simulink model "pattern3x3_training_2023clock"  (R2024a)
settings: Solver=FixedStepAuto  StartTime=0.0  StopTime=2  FixedStep=0.000005  RelTol=1e-3
model workspace (MAT data in the model file):
  part1_v1 = 1
values from neighbouring files (symbols this model uses):
  full_pattern = load('Pattern4_250.CSV')    [model_setup4.m]
  max_weight2 = 255    [model_setup4.m]
  min_weight2 = 150    [model_setup4.m]
  Th_minus_count2 = 10    [model_setup4.m]    (also in model_setup_test.m = 5)
  Th_plus_count2 = 20    [model_setup4.m]    (also in model_setup_test.m)
libraries: simulink x1
(part 1 of 9)
settings Model: Creator=ITSC  LastModifiedBy=itsc
settings SolverCC: AlgebraicLoopSolver=TrustRegion
settings OptimizationCC: ReuseModelBlockBuffer=off
settings DebuggingCC: UnconnectedInputMsg=warning  UnconnectedOutputMsg=warning  UnconnectedLineMsg=warning
settings ModelReferenceCC: EnableRefExpFcnMdlSchedulingChecks=on
settings RTWCC: GPUComputeCapability=3.5  DLArmComputeVersion=19.05

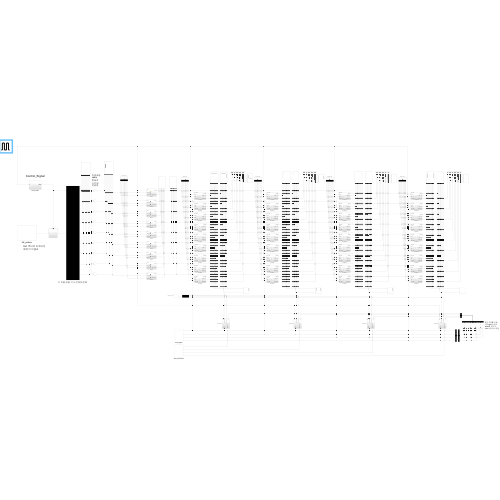
[thumbnail: Simulink's stored preview of the top-level diagram]
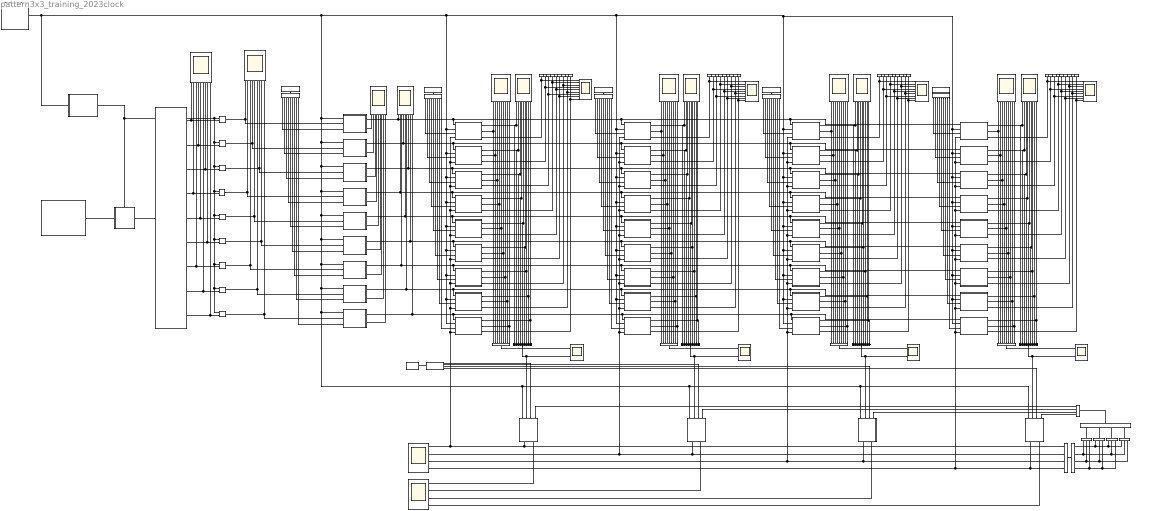
== system pattern3x3_training_2023clock ==
  note: 픽셀값을 spike 형태로 뉴런에 전달함
  note: 각 픽셀 값을 각 뉴런에게 분배
  note: 9x1 벡터로 이루어진 패턴의 픽셀값
  note: 측면 억제를 위해 다른 post 뉴런의 spike를 모아 각 post 뉴런으로 전달
  note: Control_Signal
  Bus Creator : BusCreator  Inputs=4
  Bus Creator1 : BusCreator  Inputs=4
  Bus Selector : BusSelector  OutputSignals=signal1,signal2,signal3,signal4
  Bus Selector1 : BusSelector  OutputSignals=signal1,signal2,signal3,signal4
  Demux{1..6} (6 alike) : Demux  Outputs=9
  Demux7 : Demux
  Neuron1 : Subsystem
  Neuron2 : Subsystem
  Neuron3 : Subsystem
  Neuron4 : Subsystem
  Neuron5 : Subsystem
  Neuron6 : Subsystem
  Neuron7 : Subsystem
  Neuron8 : Subsystem
  Neuron9 : Subsystem
  OR{,1..3} (4 alike) : Logic  Operator=OR  Inputs=3  IconShape=distinctive  AllPortsSameDT=off  OutDataTypeStr=boolean
  OR{8..11} (4 alike) : Logic  Operator=OR  Inputs=9  AllPortsSameDT=off  OutDataTypeStr=boolean
  Post_Neuron1 : Subsystem
  Post_Neuron2 : Subsystem
  Post_Neuron3 : Subsystem
  Post_Neuron4 : Subsystem
  Post_Spike : Scope  NumInputPorts=4
  Post_Threshold : Scope  NumInputPorts=4
  Product{1..9} (9 alike) : Product
  Pulse Generator2 : DiscretePulseGenerator  PulseType=Time based  Period=0.0001  PulseWidth=50
  Scope{,1..14,19} (16 alike) : Scope  NumInputPorts=9
  Scope{15..18} (4 alike) : Scope  NumInputPorts=2
  Subsystem1 : Subsystem
  Sum{4..7} (4 alike) : Sum  Inputs=|+++++++++
  Synapse1 : Subsystem
  Synapse10 : Subsystem
  Synapse11 : Subsystem
  Synapse12 : Subsystem
  Synapse13 : Subsystem
  Synapse14 : Subsystem
  Synapse15 : Subsystem
  Synapse16 : Subsystem
  Synapse17 : Subsystem
  Synapse18 : Subsystem
  Synapse19 : Subsystem
  Synapse2 : Subsystem
  Synapse20 : Subsystem
  Synapse21 : Subsystem
  Synapse22 : Subsystem
  Synapse23 : Subsystem
  Synapse24 : Subsystem
  Synapse25 : Subsystem
  Synapse26 : Subsystem
  Synapse27 : Subsystem
  Synapse28 : Subsystem
  Synapse29 : Subsystem
  Synapse3 : Subsystem
  Synapse30 : Subsystem
  Synapse31 : Subsystem
  Synapse32 : Subsystem
  Synapse33 : Subsystem
  Synapse34 : Subsystem
  Synapse35 : Subsystem
  Synapse36 : Subsystem
  Synapse4 : Subsystem
  Synapse5 : Subsystem
  Synapse6 : Subsystem
  Synapse7 : Subsystem
  Synapse8 : Subsystem
  Synapse9 : Subsystem
  To Workspace2 : ToWorkspace  VariableName=w1_2  SampleTime=-1
  To Workspace3 : ToWorkspace  VariableName=w2_2  SampleTime=-1
  To Workspace36 : ToWorkspace  VariableName=w1_1  SampleTime=-1
  To Workspace37 : ToWorkspace  VariableName=w2_1  SampleTime=-1
  To Workspace38 : ToWorkspace  VariableName=w3_1  SampleTime=-1
  To Workspace39 : ToWorkspace  VariableName=w4_1  SampleTime=-1
  To Workspace4 : ToWorkspace  VariableName=w3_2  SampleTime=-1
  To Workspace40 : ToWorkspace  VariableName=w5_1  SampleTime=-1
  To Workspace41 : ToWorkspace  VariableName=w6_1  SampleTime=-1
  To Workspace42 : ToWorkspace  VariableName=w7_1  SampleTime=-1
  To Workspace43 : ToWorkspace  VariableName=w8_1  SampleTime=-1
  To Workspace44 : ToWorkspace  VariableName=w9_1  SampleTime=-1
  To Workspace45 : ToWorkspace  VariableName=w9_2  SampleTime=-1
  To Workspace46 : ToWorkspace  VariableName=w1_3  SampleTime=-1
  To Workspace47 : ToWorkspace  VariableName=w2_3  SampleTime=-1
  To Workspace48 : ToWorkspace  VariableName=w3_3  SampleTime=-1
  To Workspace49 : ToWorkspace  VariableName=w4_3  SampleTime=-1
  To Workspace5 : ToWorkspace  VariableName=w4_2  SampleTime=-1
  To Workspace50 : ToWorkspace  VariableName=w5_3  SampleTime=-1
  To Workspace51 : ToWorkspace  VariableName=w6_3  SampleTime=-1
  To Workspace52 : ToWorkspace  VariableName=w7_3  SampleTime=-1
  To Workspace53 : ToWorkspace  VariableName=w8_3  SampleTime=-1
  To Workspace54 : ToWorkspace  VariableName=w9_3  SampleTime=-1
  To Workspace55 : ToWorkspace  VariableName=w1_4  SampleTime=-1
  To Workspace56 : ToWorkspace  VariableName=w2_4  SampleTime=-1
  To Workspace57 : ToWorkspace  VariableName=w3_4  SampleTime=-1
  To Workspace58 : ToWorkspace  VariableName=w4_4  SampleTime=-1
  To Workspace59 : ToWorkspace  VariableName=w5_4  SampleTime=-1
  To Workspace6 : ToWorkspace  VariableName=w5_2  SampleTime=-1
  To Workspace60 : ToWorkspace  VariableName=w6_4  SampleTime=-1
  To Workspace61 : ToWorkspace  VariableName=w7_4  SampleTime=-1
  To Workspace62 : ToWorkspace  VariableName=w8_4  SampleTime=-1
  To Workspace63 : ToWorkspace  VariableName=w9_4  SampleTime=-1
  To Workspace7 : ToWorkspace  VariableName=w6_2  SampleTime=-1
  To Workspace8 : ToWorkspace  VariableName=w7_2  SampleTime=-1
  To Workspace9 : ToWorkspace  VariableName=w8_2  SampleTime=-1
  clock_0.001 : Subsystem
  full_pattern : Constant  Value=full_pattern
  post_neuron_num : Constant  Value=[1 2 3 4]  VectorParams1D=off
  pre_neuron_num : Constant  Value=[1 2 3 4 5 6 7 8 9]  VectorParams1D=off
  synapse_num1 : Constant  Value=[1 2 3 4 5 6 7 8 9]  VectorParams1D=off
  synapse_num2 : Constant  Value=[10 11 12 13 14 15 16 17 18]  VectorParams1D=off
  synapse_num3 : Constant  Value=[19 20 21 22 23 24 25 26 27]  VectorParams1D=off
  synapse_num4 : Constant  Value=[28 29 30 31 32 33 34 35 36]  VectorParams1D=off
  wires:
  Demux1/4 -> Product3/2, Scope/2
  Demux1/5 -> Product4/2, Scope/5
  Demux1/2 -> Product1/2, Scope/4
  Demux1/6 -> Product5/2, Scope/8
  Demux1/8 -> Product7/2, Scope/6
  Subsystem1/1(y) -> Demux1/1
  Demux1/7 -> Product6/2, Scope/3
  Demux1/3 -> Product2/2, Scope/7
  Demux1/9 -> Product8/2, Scope/9
  Neuron1/1("Spike ") -> Synapse1/1(Pre_spike), Synapse10/1(Pre_spike), Synapse28/1(Pre_spike), Synapse19/1(Pre_spike), Scope9/1
  Neuron3/1("Spike ") -> Scope9/7, Synapse3/1(Pre_spike), Synapse12/1(Pre_spike), Synapse30/1(Pre_spike), Synapse21/1(Pre_spike)
  Neuron4/1("Spike ") -> Scope9/2, Synapse4/1(Pre_spike), Synapse13/1(Pre_spike), Synapse31/1(Pre_spike), Synapse22/1(Pre_spike)
  Neuron5/1("Spike ") -> Scope9/5, Synapse5/1(Pre_spike), Synapse14/1(Pre_spike), Synapse32/1(Pre_spike), Synapse23/1(Pre_spike)
  Neuron6/1("Spike ") -> Scope9/8, Synapse6/1(Pre_spike), Synapse15/1(Pre_spike), Synapse33/1(Pre_spike), Synapse24/1(Pre_spike)
  Neuron7/1("Spike ") -> Scope9/3, Synapse7/1(Pre_spike), Synapse16/1(Pre_spike), Synapse34/1(Pre_spike), Synapse25/1(Pre_spike)
  Neuron8/1("Spike ") -> Scope9/6, Synapse8/1(Pre_spike), Synapse17/1(Pre_spike), Synapse35/1(Pre_spike), Synapse26/1(Pre_spike)
  Neuron9/1("Spike ") -> Scope9/9, Synapse9/1(Pre_spike), Synapse18/1(Pre_spike), Synapse36/1(Pre_spike), Synapse27/1(Pre_spike)
  Neuron2/1("Spike ") -> Synapse2/1(Pre_spike), Synapse11/1(Pre_spike), Synapse29/1(Pre_spike), Synapse20/1(Pre_spike), Scope9/4
  OR8/1 -> Scope15/1
  Sum5/1 -> Post_Neuron1/2(Input_potential), Scope15/2
  Synapse8/2(Spike_out) -> Scope4/8, OR8/8
  Synapse7/2(Spike_out) -> Scope4/7, OR8/7
  Synapse6/2(Spike_out) -> Scope4/6, OR8/6
  Synapse4/1(Weight) -> Scope8/4, Sum5/4
  Synapse4/2(Spike_out) -> Scope4/4, OR8/4
  Synapse3/1(Weight) -> Scope8/3, Sum5/3
  Synapse3/2(Spike_out) -> Scope4/3, OR8/3
  Synapse2/2(Spike_out) -> Scope4/2, OR8/2
  Synapse9/2(Spike_out) -> Scope4/9, OR8/9
  Synapse1/2(Spike_out) -> Scope4/1, OR8/1
  Synapse5/2(Spike_out) -> Scope4/5, OR8/5
  Synapse7/1(Weight) -> Scope8/7, Sum5/7
  Synapse8/1(Weight) -> Scope8/8, Sum5/8
  Synapse9/1(Weight) -> Scope8/9, Sum5/9
  Neuron1/2(threshold_view) -> Scope7/1
  Neuron2/2(threshold_view) -> Scope7/2
  Neuron3/2(threshold_view) -> Scope7/3
  Neuron4/2(threshold_view) -> Scope7/4
  Neuron5/2(threshold_view) -> Scope7/5
  Neuron6/2(threshold_view) -> Scope7/6
  Neuron7/2(threshold_view) -> Scope7/7
  Neuron8/2(threshold_view) -> Scope7/8
  Neuron9/2(threshold_view) -> Scope7/9
  synapse_num1/1 -> Demux2/1
  Synapse5/1(Weight) -> Scope8/5, Sum5/5
  Synapse6/1(Weight) -> Scope8/6, Sum5/6
  Demux2/1 -> Synapse1/3(addr)
  Demux2/2 -> Synapse2/3(addr)
  Demux2/3 -> Synapse3/3(addr)
  Demux2/4 -> Synapse4/3(addr)
  Demux2/5 -> Synapse5/3(addr)
  Demux2/6 -> Synapse6/3(addr)
  Demux2/7 -> Synapse7/3(addr)
  Demux2/8 -> Synapse8/3(addr)
  Demux2/9 -> Synapse9/3(addr)
  Demux3/5 -> Synapse14/3(addr)
  Demux3/1 -> Synapse10/3(addr)
  Demux3/6 -> Synapse15/3(addr)
  Demux3/7 -> Synapse16/3(addr)
  Demux3/8 -> Synapse17/3(addr)
  Demux3/2 -> Synapse11/3(addr)
  Demux3/3 -> Synapse12/3(addr)
  Demux3/4 -> Synapse13/3(addr)
  Demux3/9 -> Synapse18/3(addr)
  synapse_num2/1 -> Demux3/1
  Demux4/1 -> Synapse19/3(addr)
  Demux4/8 -> Synapse26/3(addr)
  Demux4/7 -> Synapse25/3(addr)
  synapse_num3/1 -> Demux4/1
  Demux4/2 -> Synapse20/3(addr)
  Demux4/5 -> Synapse23/3(addr)
  Demux4/9 -> Synapse27/3(addr)
  Demux4/4 -> Synapse22/3(addr)
  Demux4/3 -> Synapse21/3(addr)
  Demux4/6 -> Synapse24/3(addr)
  Demux5/5 -> Synapse32/3(addr)
  Demux5/1 -> Synapse28/3(addr)
  Demux5/6 -> Synapse33/3(addr)
  Demux5/7 -> Synapse34/3(addr)
  Demux5/8 -> Synapse35/3(addr)
  Demux5/2 -> Synapse29/3(addr)
  Demux5/3 -> Synapse30/3(addr)
  Demux5/4 -> Synapse31/3(addr)
  Demux5/9 -> Synapse36/3(addr)
  synapse_num4/1 -> Demux5/1
  Post_Neuron1/1(Spike) -> Synapse9/4(Post_spike), Synapse8/4(Post_spike), Synapse7/4(Post_spike), Synapse6/4(Post_spike), Synapse5/4(Post_spike), Synapse4/4(Post_spike), Synapse3/4(Post_spike), Synapse2/4(Post_spike), Synapse1/4(Post_spike), Post_Spike/1, Bus Creator/1
  Post_Neuron2/1(Spike) -> Synapse18/4(Post_spike), Synapse17/4(Post_spike), Synapse16/4(Post_spike), Synapse15/4(Post_spike), Synapse14/4(Post_spike), Synapse13/4(Post_spike), Synapse12/4(Post_spike), Synapse11/4(Post_spike), Synapse10/4(Post_spike), Post_Spike/2, Bus Creator/2
  Post_Neuron3/1(Spike) -> Synapse27/4(Post_spike), Synapse26/4(Post_spike), Synapse25/4(Post_spike), Synapse24/4(Post_spike), Synapse23/4(Post_spike), Synapse22/4(Post_spike), Synapse21/4(Post_spike), Synapse19/4(Post_spike), Synapse20/4(Post_spike), Post_Spike/3, Bus Creator/3
  Post_Neuron1/2(threshold_view) -> Post_Threshold/1
  Post_Neuron2/2(threshold_view) -> Post_Threshold/2
  Post_Neuron3/2(threshold_view) -> Post_Threshold/3
  Post_Neuron4/2(threshold_view) -> Post_Threshold/4
  Post_Neuron4/1(Spike) -> Synapse36/4(Post_spike), Synapse35/4(Post_spike), Synapse34/4(Post_spike), Synapse33/4(Post_spike), Synapse32/4(Post_spike), Synapse31/4(Post_spike), Synapse30/4(Post_spike), Synapse29/4(Post_spike), Synapse28/4(Post_spike), Post_Spike/4, Bus Creator/4
  Synapse6/3(Weight_out) -> Scope11/8, To Workspace41/1
  Synapse9/3(Weight_out) -> Scope11/9, To Workspace44/1
  Synapse7/3(Weight_out) -> Scope11/3, To Workspace42/1
  Synapse1/3(Weight_out) -> Scope11/1, To Workspace36/1
  Synapse4/3(Weight_out) -> Scope11/2, To Workspace39/1
  Synapse8/3(Weight_out) -> Scope11/6, To Workspace43/1
  Synapse2/3(Weight_out) -> Scope11/4, To Workspace37/1
  Synapse3/3(Weight_out) -> Scope11/7, To Workspace38/1
  Synapse15/2(Spike_out) -> Scope5/6, OR9/6
  Synapse12/2(Spike_out) -> Scope5/3, OR9/3
  Synapse18/2(Spike_out) -> Scope5/9, OR9/9
  Synapse13/2(Spike_out) -> Scope5/4, OR9/4
  Synapse10/2(Spike_out) -> Scope5/1, OR9/1
  Synapse11/2(Spike_out) -> Scope5/2, OR9/2
  Synapse16/2(Spike_out) -> Scope5/7, OR9/7
  Synapse14/2(Spike_out) -> Scope5/5, OR9/5
  Synapse17/2(Spike_out) -> Scope5/8, OR9/8
  Synapse24/2(Spike_out) -> Scope6/6, OR10/6
  Synapse21/2(Spike_out) -> Scope6/3, OR10/3
  Synapse27/2(Spike_out) -> Scope6/9, OR10/9
  Synapse22/2(Spike_out) -> Scope6/4, OR10/4
  Synapse19/2(Spike_out) -> Scope6/1, OR10/1
  Synapse20/2(Spike_out) -> Scope6/2, OR10/2
  Synapse25/2(Spike_out) -> Scope6/7, OR10/7
  Synapse23/2(Spike_out) -> Scope6/5, OR10/5
  Synapse26/2(Spike_out) -> Scope6/8, OR10/8
  Synapse33/2(Spike_out) -> Scope10/6, OR11/6
  Synapse30/2(Spike_out) -> Scope10/3, OR11/3
  Synapse36/2(Spike_out) -> Scope10/9, OR11/9
  Synapse31/2(Spike_out) -> Scope10/4, OR11/4
  Synapse28/2(Spike_out) -> Scope10/1, OR11/1
  Synapse29/2(Spike_out) -> Scope10/2, OR11/2
  Synapse34/2(Spike_out) -> Scope10/7, OR11/7
  Synapse32/2(Spike_out) -> Scope10/5, OR11/5
  Synapse35/2(Spike_out) -> Scope10/8, OR11/8
  Synapse5/3(Weight_out) -> Scope11/5, To Workspace40/1
  Synapse16/3(Weight_out) -> Scope12/3, To Workspace8/1
  Synapse12/3(Weight_out) -> Scope12/7, To Workspace4/1
  Synapse11/3(Weight_out) -> Scope12/4, To Workspace3/1
  Synapse15/3(Weight_out) -> Scope12/8, To Workspace7/1
  Synapse14/3(Weight_out) -> Scope12/5, To Workspace6/1
  Synapse13/3(Weight_out) -> Scope12/2, To Workspace5/1
  Synapse17/3(Weight_out) -> Scope12/6, To Workspace9/1
  Synapse10/3(Weight_out) -> Scope12/1, To Workspace2/1
  Synapse18/3(Weight_out) -> Scope12/9, To Workspace45/1
  Synapse25/3(Weight_out) -> Scope13/3, To Workspace52/1
  Synapse21/3(Weight_out) -> Scope13/7, To Workspace48/1
  Synapse20/3(Weight_out) -> Scope13/4, To Workspace47/1
  Synapse24/3(Weight_out) -> Scope13/8, To Workspace51/1
  Synapse23/3(Weight_out) -> To Workspace50/1, Scope13/5
  Synapse22/3(Weight_out) -> Scope13/2, To Workspace49/1
  Synapse26/3(Weight_out) -> Scope13/6, To Workspace53/1
  Synapse19/3(Weight_out) -> To Workspace46/1, Scope13/1
  Synapse27/3(Weight_out) -> To Workspace54/1, Scope13/9
  Synapse34/3(Weight_out) -> Scope14/3, To Workspace61/1
  Synapse30/3(Weight_out) -> Scope14/7, To Workspace57/1
  Synapse29/3(Weight_out) -> Scope14/4, To Workspace56/1
  Synapse33/3(Weight_out) -> Scope14/8, To Workspace60/1
  Synapse32/3(Weight_out) -> Scope14/5, To Workspace59/1
  Synapse31/3(Weight_out) -> Scope14/2, To Workspace58/1
  Synapse35/3(Weight_out) -> Scope14/6, To Workspace62/1
  Synapse28/3(Weight_out) -> Scope14/1, To Workspace55/1
  Synapse36/3(Weight_out) -> Scope14/9, To Workspace63/1
  OR9/1 -> Scope16/1
  Sum4/1 -> Post_Neuron2/2(Input_potential), Scope16/2
  OR10/1 -> Scope17/1
  Sum6/1 -> Post_Neuron3/2(Input_potential), Scope17/2
  Sum7/1 -> Post_Neuron4/2(Input_potential), Scope18/2
  OR11/1 -> Scope18/1
  Synapse1/1(Weight) -> Scope8/1, Sum5/1
  Synapse2/1(Weight) -> Scope8/2, Sum5/2
  Synapse14/1(Weight) -> Scope1/5, Sum4/5
  Synapse12/1(Weight) -> Scope1/3, Sum4/3
  Synapse13/1(Weight) -> Scope1/4, Sum4/4
  Synapse10/1(Weight) -> Scope1/1, Sum4/1
  Synapse15/1(Weight) -> Scope1/6, Sum4/6
  Synapse18/1(Weight) -> Scope1/9, Sum4/9
  Synapse17/1(Weight) -> Scope1/8, Sum4/8
  Synapse16/1(Weight) -> Scope1/7, Sum4/7
  Synapse11/1(Weight) -> Scope1/2, Sum4/2
  Synapse23/1(Weight) -> Scope2/5, Sum6/5
  Synapse21/1(Weight) -> Scope2/3, Sum6/3
  Synapse22/1(Weight) -> Scope2/4, Sum6/4
  Synapse19/1(Weight) -> Scope2/1, Sum6/1
  Synapse24/1(Weight) -> Scope2/6, Sum6/6
  Synapse27/1(Weight) -> Scope2/9, Sum6/9
  Synapse26/1(Weight) -> Scope2/8, Sum6/8
  Synapse25/1(Weight) -> Scope2/7, Sum6/7
  Synapse20/1(Weight) -> Scope2/2, Sum6/2
  Synapse32/1(Weight) -> Scope3/5, Sum7/5
  Synapse30/1(Weight) -> Scope3/3, Sum7/3
  Synapse31/1(Weight) -> Scope3/4, Sum7/4
  Synapse28/1(Weight) -> Scope3/1, Sum7/1
  Synapse33/1(Weight) -> Scope3/6, Sum7/6
  Synapse36/1(Weight) -> Scope3/9, Sum7/9
  Synapse35/1(Weight) -> Scope3/8, Sum7/8
  Synapse34/1(Weight) -> Scope3/7, Sum7/7
  Synapse29/1(Weight) -> Scope3/2, Sum7/2
  clock_0.001/1(clock) -> Subsystem1/Trigger, Product3/1, Product4/1, Product8/1, Product7/1, Product6/1, Product5/1, Product2/1, Product1/1, Product9/1
  Demux1/1 -> Product9/2, Scope/1
  Demux6/5 -> Neuron5/3(neuron_num)
  Demux6/6 -> Neuron6/3(neuron_num)
  Demux6/7 -> Neuron7/3(neuron_num)
  Demux6/4 -> Neuron4/3(neuron_num)
  Demux6/3 -> Neuron3/3(neuron_num)
  Demux6/2 -> Neuron2/3(neuron_num)
  Demux6/9 -> Neuron9/3(neuron_num)
  Demux6/8 -> Neuron8/3(neuron_num)
  Demux6/1 -> Neuron1/3(neuron_num)
  pre_neuron_num/1 -> Demux6/1
  post_neuron_num/1 -> Demux7/1
  Demux7/1 -> Post_Neuron1/3(neuron_num)
  Demux7/2 -> Post_Neuron2/3(neuron_num)
  Demux7/3 -> Post_Neuron3/3(neuron_num)
  Demux7/4 -> Post_Neuron4/3(neuron_num)
  Bus Creator/1 -> Bus Selector/1
  Bus Selector/2 -> OR3/2, OR2/2, OR/1  "<signal2>"
  Bus Selector/3 -> OR3/3, OR1/2, OR/2  "<signal3>"
  Bus Selector/4 -> OR2/3, OR1/3, OR/3  "<signal4>"
  Bus Selector/1 -> OR3/1, OR2/1, OR1/1  "<signal1>"
  OR/1 -> Bus Creator1/1
  OR3/1 -> Bus Creator1/4
  OR2/1 -> Bus Creator1/3
  OR1/1 -> Bus Creator1/2
  Bus Creator1/1 -> Bus Selector1/1
  Bus Selector1/1 -> Post_Neuron1/4(wta)  "<signal1>"
  Bus Selector1/2 -> Post_Neuron2/4(wta)  "<signal2>"
  Bus Selector1/3 -> Post_Neuron3/4(wta)  "<signal3>"
  Bus Selector1/4 -> Post_Neuron4/4(wta)  "<signal4>"
  full_pattern/1 -> Subsystem1/1(data)
  Product1/1 -> Neuron2/2(Input_potential), Scope19/4
  Product5/1 -> Neuron6/2(Input_potential), Scope19/8
  Product2/1 -> Neuron3/2(Input_potential), Scope19/7
  Product4/1 -> Neuron5/2(Input_potential), Scope19/5
  Product7/1 -> Neuron8/2(Input_potential), Scope19/6
  Product3/1 -> Neuron4/2(Input_potential), Scope19/2
  Product6/1 -> Neuron7/2(Input_potential), Scope19/3
  Product8/1 -> Neuron9/2(Input_potential), Scope19/9
  Product9/1 -> Neuron1/2(Input_potential), Scope19/1
  Pulse Generator2/1 -> clock_0.001/1(In1), Neuron1/1(clock), Neuron2/1(clock), Neuron3/1(clock), Neuron4/1(clock), Neuron5/1(clock), Neuron6/1(clock), Neuron7/1(clock), Neuron8/1(clock), Neuron9/1(clock), Post_Neuron2/1(clock), Post_Neuron4/1(clock), Post_Neuron3/1(clock), Post_Neuron1/1(clock), Synapse28/2(clock), Synapse29/2(clock), Synapse30/2(clock), Synapse31/2(clock), Synapse32/2(clock), Synapse33/2(clock), Synapse34/2(clock), Synapse36/2(clock), Synapse35/2(clock), Synapse19/2(clock), Synapse20/2(clock), Synapse21/2(clock), Synapse22/2(clock), Synapse23/2(clock), Synapse24/2(clock), Synapse25/2(clock), Synapse27/2(clock), Synapse26/2(clock), Synapse10/2(clock), Synapse11/2(clock), Synapse12/2(clock), Synapse13/2(clock), Synapse14/2(clock), Synapse15/2(clock), Synapse16/2(clock), Synapse18/2(clock), Synapse17/2(clock), Synapse2/2(clock), Synapse3/2(clock), Synapse4/2(clock), Synapse5/2(clock), Synapse6/2(clock), Synapse7/2(clock), Synapse9/2(clock), Synapse8/2(clock), Synapse1/2(clock)

== system pattern3x3_training_2023clock/Neuron1 ==
  note: Membrane potential part
  note: Input potential이 추가로 들어오기 전에는 이전
      | membrane state를 유지해야 하기 때문에 Trigger 사용
  note: Output 스파이크 빈도에 따라 Threshold 조절
  note: membrane potential>=threshold
  note: membrane potential
      | - threshold
  note: 뉴런 번호
  note: membrane potential<threshold
  note: membrane potential - threshold >= 0 일때 spike=1
  note: Threshold part
  note: Spike part
  note: membrane state
      | - threshold
  clock : Inport
  Input_potential : Inport  Port=2  OutDataTypeStr=double
  neuron_num : Inport  Port=3  OutDataTypeStr=double
  Clock4 : Subsystem
  Delay : Delay  DelayLength=1  InitialCondition=0
  From Workspace4 : FromWorkspace  VariableName=threshold_pre
  MATLAB Function3 : MATLAB Function  TreatAsAtomicUnit=on
  MATLAB Function4 : MATLAB Function  TreatAsAtomicUnit=on
  MATLAB Function5 : MATLAB Function  TreatAsAtomicUnit=on
  Memory2 : Memory
  Scope4 : Scope  NumInputPorts=5
  Scope9 : Scope  NumInputPorts=6
  Subsystem2 : Subsystem
  Subsystem3 : Subsystem
  Subtract2 : Sum  Inputs=+-
  Subtract3 : Sum  Inputs=+-
  Switch1 : Switch  SaturateOnIntegerOverflow=off  InputSameDT=off
  spike_generator1 : Subsystem
  "Spike " : Outport  VectorParamsAs1DForOutWhenUnconnected=off
  threshold_view : Outport  Port=2
  wires:
  Switch1/1 -> Delay/1, Subtract2/1, Scope9/1
  Subtract2/1 -> Scope9/3, MATLAB Function3/1(u)
  MATLAB Function3/1(y) -> Memory2/1, Scope9/4
  Clock4/1(T) -> Scope4/3, MATLAB Function5/1(t), MATLAB Function4/2(t)
  Subsystem3/1(Threshold) -> Subtract2/2, Scope9/2, Subtract3/2, threshold_view/1
  neuron_num/1 -> Subsystem3/3(neuron_num)
  From Workspace4/1 -> Subsystem3/2(initial_threshold)
  MATLAB Function5/1(membrane_potential) -> Scope4/4, Switch1/1
  MATLAB Function4/1(membrane_potential) -> Switch1/3, Scope4/5
  Subsystem2/1(membrane_state) -> MATLAB Function4/1(membrane_state), Subtract3/1, Scope4/2, MATLAB Function5/2(membrane_state)
  spike_generator1/1(spike) -> "Spike "/1, Scope9/6, Subsystem3/1(spike)
  Input_potential/1 -> Subsystem2/1(Input potential), Subsystem2/Trigger, Scope4/1, Clock4/2("Reset ")
  Subtract3/1 -> Switch1/2
  Memory2/1 -> Scope9/5, spike_generator1/1(1)
  Delay/1 -> Subsystem2/2(before_Potential)
  clock/1 -> Subsystem3/4(clock), Clock4/1(clock)

== system pattern3x3_training_2023clock/Neuron2 ==
  note: Membrane potential part
  note: Input potential이 추가로 들어오기 전에는 이전
      | membrane state를 유지해야 하기 때문에 Trigger 사용
  note: Output 스파이크 빈도에 따라 Threshold 조절
  note: membrane potential>=threshold
  note: membrane potential
      | - threshold
  note: 뉴런 번호
  note: membrane potential<threshold
  note: membrane potential - threshold >= 0 일때 spike=1
  note: Threshold part
  note: Spike part
  note: membrane state
      | - threshold
  clock : Inport
  Input_potential : Inport  Port=2  OutDataTypeStr=double
  neuron_num : Inport  Port=3  OutDataTypeStr=double
  Clock4 : Subsystem
  Delay : Delay  DelayLength=1  InitialCondition=0
  From Workspace4 : FromWorkspace  VariableName=threshold_pre
  MATLAB Function3 : MATLAB Function  TreatAsAtomicUnit=on
  MATLAB Function4 : MATLAB Function  TreatAsAtomicUnit=on
  MATLAB Function5 : MATLAB Function  TreatAsAtomicUnit=on
  Memory2 : Memory
  Scope4 : Scope  NumInputPorts=5
  Scope9 : Scope  NumInputPorts=6
  Subsystem2 : Subsystem
  Subsystem3 : Subsystem
  Subtract2 : Sum  Inputs=+-
  Subtract3 : Sum  Inputs=+-
  Switch1 : Switch  SaturateOnIntegerOverflow=off  InputSameDT=off
  spike_generator1 : Subsystem
  "Spike " : Outport  VectorParamsAs1DForOutWhenUnconnected=off
  threshold_view : Outport  Port=2
  wires:
  Switch1/1 -> Delay/1, Subtract2/1, Scope9/1
  Subtract2/1 -> Scope9/3, MATLAB Function3/1(u)
  MATLAB Function3/1(y) -> Memory2/1, Scope9/4
  Clock4/1(T) -> Scope4/3, MATLAB Function5/1(t), MATLAB Function4/2(t)
  Subsystem3/1(Threshold) -> Subtract2/2, Scope9/2, Subtract3/2, threshold_view/1
  neuron_num/1 -> Subsystem3/3(neuron_num)
  From Workspace4/1 -> Subsystem3/2(initial_threshold)
  MATLAB Function5/1(membrane_potential) -> Scope4/4, Switch1/1
  MATLAB Function4/1(membrane_potential) -> Switch1/3, Scope4/5
  Subsystem2/1(membrane_state) -> MATLAB Function4/1(membrane_state), Subtract3/1, Scope4/2, MATLAB Function5/2(membrane_state)
  spike_generator1/1(spike) -> "Spike "/1, Scope9/6, Subsystem3/1(spike)
  Input_potential/1 -> Subsystem2/1(Input potential), Subsystem2/Trigger, Scope4/1, Clock4/2("Reset ")
  Subtract3/1 -> Switch1/2
  Memory2/1 -> Scope9/5, spike_generator1/1(1)
  Delay/1 -> Subsystem2/2(before_Potential)
  clock/1 -> Subsystem3/4(clock), Clock4/1(clock)

== system pattern3x3_training_2023clock/Neuron3 ==
  note: Membrane potential part
  note: Input potential이 추가로 들어오기 전에는 이전
      | membrane state를 유지해야 하기 때문에 Trigger 사용
  note: Output 스파이크 빈도에 따라 Threshold 조절
  note: membrane potential>=threshold
  note: membrane potential
      | - threshold
  note: 뉴런 번호
  note: membrane potential<threshold
  note: membrane potential - threshold >= 0 일때 spike=1
  note: Threshold part
  note: Spike part
  note: membrane state
      | - threshold
  clock : Inport
  Input_potential : Inport  Port=2  OutDataTypeStr=double
  neuron_num : Inport  Port=3  OutDataTypeStr=double
  Clock4 : Subsystem
  Delay : Delay  DelayLength=1  InitialCondition=0
  From Workspace4 : FromWorkspace  VariableName=threshold_pre
  MATLAB Function3 : MATLAB Function  TreatAsAtomicUnit=on
  MATLAB Function4 : MATLAB Function  TreatAsAtomicUnit=on
  MATLAB Function5 : MATLAB Function  TreatAsAtomicUnit=on
  Memory2 : Memory
  Scope4 : Scope  NumInputPorts=5
  Scope9 : Scope  NumInputPorts=6
  Subsystem2 : Subsystem
  Subsystem3 : Subsystem
  Subtract2 : Sum  Inputs=+-
  Subtract3 : Sum  Inputs=+-
  Switch1 : Switch  SaturateOnIntegerOverflow=off  InputSameDT=off
  spike_generator1 : Subsystem
  "Spike " : Outport  VectorParamsAs1DForOutWhenUnconnected=off
  threshold_view : Outport  Port=2
  wires:
  Switch1/1 -> Delay/1, Subtract2/1, Scope9/1
  Subtract2/1 -> Scope9/3, MATLAB Function3/1(u)
  MATLAB Function3/1(y) -> Memory2/1, Scope9/4
  Clock4/1(T) -> Scope4/3, MATLAB Function5/1(t), MATLAB Function4/2(t)
  Subsystem3/1(Threshold) -> Subtract2/2, Scope9/2, Subtract3/2, threshold_view/1
  neuron_num/1 -> Subsystem3/3(neuron_num)
  From Workspace4/1 -> Subsystem3/2(initial_threshold)
  MATLAB Function5/1(membrane_potential) -> Scope4/4, Switch1/1
  MATLAB Function4/1(membrane_potential) -> Switch1/3, Scope4/5
  Subsystem2/1(membrane_state) -> MATLAB Function4/1(membrane_state), Subtract3/1, Scope4/2, MATLAB Function5/2(membrane_state)
  spike_generator1/1(spike) -> "Spike "/1, Scope9/6, Subsystem3/1(spike)
  Input_potential/1 -> Subsystem2/1(Input potential), Subsystem2/Trigger, Scope4/1, Clock4/2("Reset ")
  Subtract3/1 -> Switch1/2
  Memory2/1 -> Scope9/5, spike_generator1/1(1)
  Delay/1 -> Subsystem2/2(before_Potential)
  clock/1 -> Subsystem3/4(clock), Clock4/1(clock)

== system pattern3x3_training_2023clock/Neuron4 ==
  note: Membrane potential part
  note: Input potential이 추가로 들어오기 전에는 이전
      | membrane state를 유지해야 하기 때문에 Trigger 사용
  note: Output 스파이크 빈도에 따라 Threshold 조절
  note: membrane potential>=threshold
  note: membrane potential
      | - threshold
  note: 뉴런 번호
  note: membrane potential<threshold
  note: membrane potential - threshold >= 0 일때 spike=1
  note: Threshold part
  note: Spike part
  note: membrane state
      | - threshold
  clock : Inport
  Input_potential : Inport  Port=2  OutDataTypeStr=double
  neuron_num : Inport  Port=3  OutDataTypeStr=double
  Clock4 : Subsystem
  Delay : Delay  DelayLength=1  InitialCondition=0
  From Workspace4 : FromWorkspace  VariableName=threshold_pre
  MATLAB Function3 : MATLAB Function  TreatAsAtomicUnit=on
  MATLAB Function4 : MATLAB Function  TreatAsAtomicUnit=on
  MATLAB Function5 : MATLAB Function  TreatAsAtomicUnit=on
  Memory2 : Memory
  Scope4 : Scope  NumInputPorts=5
  Scope9 : Scope  NumInputPorts=6
  Subsystem2 : Subsystem
  Subsystem3 : Subsystem
  Subtract2 : Sum  Inputs=+-
  Subtract3 : Sum  Inputs=+-
  Switch1 : Switch  SaturateOnIntegerOverflow=off  InputSameDT=off
  spike_generator1 : Subsystem
  "Spike " : Outport  VectorParamsAs1DForOutWhenUnconnected=off
  threshold_view : Outport  Port=2
  wires:
  Switch1/1 -> Delay/1, Subtract2/1, Scope9/1
  Subtract2/1 -> Scope9/3, MATLAB Function3/1(u)
  MATLAB Function3/1(y) -> Memory2/1, Scope9/4
  Clock4/1(T) -> Scope4/3, MATLAB Function5/1(t), MATLAB Function4/2(t)
  Subsystem3/1(Threshold) -> Subtract2/2, Scope9/2, Subtract3/2, threshold_view/1
  neuron_num/1 -> Subsystem3/3(neuron_num)
  From Workspace4/1 -> Subsystem3/2(initial_threshold)
  MATLAB Function5/1(membrane_potential) -> Scope4/4, Switch1/1
  MATLAB Function4/1(membrane_potential) -> Switch1/3, Scope4/5
  Subsystem2/1(membrane_state) -> MATLAB Function4/1(membrane_state), Subtract3/1, Scope4/2, MATLAB Function5/2(membrane_state)
  spike_generator1/1(spike) -> "Spike "/1, Scope9/6, Subsystem3/1(spike)
  Input_potential/1 -> Subsystem2/1(Input potential), Subsystem2/Trigger, Scope4/1, Clock4/2("Reset ")
  Subtract3/1 -> Switch1/2
  Memory2/1 -> Scope9/5, spike_generator1/1(1)
  Delay/1 -> Subsystem2/2(before_Potential)
  clock/1 -> Subsystem3/4(clock), Clock4/1(clock)

== system pattern3x3_training_2023clock/Neuron5 ==
  note: Membrane potential part
  note: Input potential이 추가로 들어오기 전에는 이전
      | membrane state를 유지해야 하기 때문에 Trigger 사용
  note: Output 스파이크 빈도에 따라 Threshold 조절
  note: membrane potential>=threshold
  note: membrane potential
      | - threshold
  note: 뉴런 번호
  note: membrane potential<threshold
  note: membrane potential - threshold >= 0 일때 spike=1
  note: Threshold part
  note: Spike part
  note: membrane state
      | - threshold
  clock : Inport
  Input_potential : Inport  Port=2  OutDataTypeStr=double
  neuron_num : Inport  Port=3  OutDataTypeStr=double
  Clock4 : Subsystem
  Delay : Delay  DelayLength=1  InitialCondition=0
  From Workspace4 : FromWorkspace  VariableName=threshold_pre
  MATLAB Function3 : MATLAB Function  TreatAsAtomicUnit=on
  MATLAB Function4 : MATLAB Function  TreatAsAtomicUnit=on
  MATLAB Function5 : MATLAB Function  TreatAsAtomicUnit=on
  Memory2 : Memory
  Scope4 : Scope  NumInputPorts=5
  Scope9 : Scope  NumInputPorts=6
  Subsystem2 : Subsystem
  Subsystem3 : Subsystem
  Subtract2 : Sum  Inputs=+-
  Subtract3 : Sum  Inputs=+-
  Switch1 : Switch  SaturateOnIntegerOverflow=off  InputSameDT=off
  spike_generator1 : Subsystem
  "Spike " : Outport  VectorParamsAs1DForOutWhenUnconnected=off
  threshold_view : Outport  Port=2
  wires:
  Switch1/1 -> Delay/1, Subtract2/1, Scope9/1
  Subtract2/1 -> Scope9/3, MATLAB Function3/1(u)
  MATLAB Function3/1(y) -> Memory2/1, Scope9/4
  Clock4/1(T) -> Scope4/3, MATLAB Function5/1(t), MATLAB Function4/2(t)
  Subsystem3/1(Threshold) -> Subtract2/2, Scope9/2, Subtract3/2, threshold_view/1
  neuron_num/1 -> Subsystem3/3(neuron_num)
  From Workspace4/1 -> Subsystem3/2(initial_threshold)
  MATLAB Function5/1(membrane_potential) -> Scope4/4, Switch1/1
  MATLAB Function4/1(membrane_potential) -> Switch1/3, Scope4/5
  Subsystem2/1(membrane_state) -> MATLAB Function4/1(membrane_state), Subtract3/1, Scope4/2, MATLAB Function5/2(membrane_state)
  spike_generator1/1(spike) -> "Spike "/1, Scope9/6, Subsystem3/1(spike)
  Input_potential/1 -> Subsystem2/1(Input potential), Subsystem2/Trigger, Scope4/1, Clock4/2("Reset ")
  Subtract3/1 -> Switch1/2
  Memory2/1 -> Scope9/5, spike_generator1/1(1)
  Delay/1 -> Subsystem2/2(before_Potential)
  clock/1 -> Subsystem3/4(clock), Clock4/1(clock)

== system pattern3x3_training_2023clock/Neuron6 ==
  note: Membrane potential part
  note: Input potential이 추가로 들어오기 전에는 이전
      | membrane state를 유지해야 하기 때문에 Trigger 사용
  note: Output 스파이크 빈도에 따라 Threshold 조절
  note: membrane potential>=threshold
  note: membrane potential
      | - threshold
  note: 뉴런 번호
  note: membrane potential<threshold
  note: membrane potential - threshold >= 0 일때 spike=1
  note: Threshold part
  note: Spike part
  note: membrane state
      | - threshold
  clock : Inport
  Input_potential : Inport  Port=2  OutDataTypeStr=double
  neuron_num : Inport  Port=3  OutDataTypeStr=double
  Clock4 : Subsystem
  Delay : Delay  DelayLength=1  InitialCondition=0
  From Workspace4 : FromWorkspace  VariableName=threshold_pre
  MATLAB Function3 : MATLAB Function  TreatAsAtomicUnit=on
  MATLAB Function4 : MATLAB Function  TreatAsAtomicUnit=on
  MATLAB Function5 : MATLAB Function  TreatAsAtomicUnit=on
  Memory2 : Memory
  Scope4 : Scope  NumInputPorts=5
  Scope9 : Scope  NumInputPorts=6
  Subsystem2 : Subsystem
  Subsystem3 : Subsystem
  Subtract2 : Sum  Inputs=+-
  Subtract3 : Sum  Inputs=+-
  Switch1 : Switch  SaturateOnIntegerOverflow=off  InputSameDT=off
  spike_generator1 : Subsystem
  "Spike " : Outport  VectorParamsAs1DForOutWhenUnconnected=off
  threshold_view : Outport  Port=2
  wires:
  Switch1/1 -> Delay/1, Subtract2/1, Scope9/1
  Subtract2/1 -> Scope9/3, MATLAB Function3/1(u)
  MATLAB Function3/1(y) -> Memory2/1, Scope9/4
  Clock4/1(T) -> Scope4/3, MATLAB Function5/1(t), MATLAB Function4/2(t)
  Subsystem3/1(Threshold) -> Subtract2/2, Scope9/2, Subtract3/2, threshold_view/1
  neuron_num/1 -> Subsystem3/3(neuron_num)
  From Workspace4/1 -> Subsystem3/2(initial_threshold)
  MATLAB Function5/1(membrane_potential) -> Scope4/4, Switch1/1
  MATLAB Function4/1(membrane_potential) -> Switch1/3, Scope4/5
  Subsystem2/1(membrane_state) -> MATLAB Function4/1(membrane_state), Subtract3/1, Scope4/2, MATLAB Function5/2(membrane_state)
  spike_generator1/1(spike) -> "Spike "/1, Scope9/6, Subsystem3/1(spike)
  Input_potential/1 -> Subsystem2/1(Input potential), Subsystem2/Trigger, Scope4/1, Clock4/2("Reset ")
  Subtract3/1 -> Switch1/2
  Memory2/1 -> Scope9/5, spike_generator1/1(1)
  Delay/1 -> Subsystem2/2(before_Potential)
  clock/1 -> Subsystem3/4(clock), Clock4/1(clock)

== system pattern3x3_training_2023clock/Neuron7 ==
  note: Membrane potential part
  note: Input potential이 추가로 들어오기 전에는 이전
      | membrane state를 유지해야 하기 때문에 Trigger 사용
  note: Output 스파이크 빈도에 따라 Threshold 조절
  note: membrane potential>=threshold
  note: membrane potential
      | - threshold
  note: 뉴런 번호
  note: membrane potential<threshold
  note: membrane potential - threshold >= 0 일때 spike=1
  note: Threshold part
  note: Spike part
  note: membrane state
      | - threshold
  clock : Inport
  Input_potential : Inport  Port=2  OutDataTypeStr=double
  neuron_num : Inport  Port=3  OutDataTypeStr=double
  Clock4 : Subsystem
  Delay : Delay  DelayLength=1  InitialCondition=0
  From Workspace4 : FromWorkspace  VariableName=threshold_pre
  MATLAB Function3 : MATLAB Function  TreatAsAtomicUnit=on
  MATLAB Function4 : MATLAB Function  TreatAsAtomicUnit=on
  MATLAB Function5 : MATLAB Function  TreatAsAtomicUnit=on
  Memory2 : Memory
  Scope4 : Scope  NumInputPorts=5
  Scope9 : Scope  NumInputPorts=6
  Subsystem2 : Subsystem
  Subsystem3 : Subsystem
  Subtract2 : Sum  Inputs=+-
  Subtract3 : Sum  Inputs=+-
  Switch1 : Switch  SaturateOnIntegerOverflow=off  InputSameDT=off
  spike_generator1 : Subsystem
  "Spike " : Outport  VectorParamsAs1DForOutWhenUnconnected=off
  threshold_view : Outport  Port=2
  wires:
  Switch1/1 -> Delay/1, Subtract2/1, Scope9/1
  Subtract2/1 -> Scope9/3, MATLAB Function3/1(u)
  MATLAB Function3/1(y) -> Memory2/1, Scope9/4
  Clock4/1(T) -> Scope4/3, MATLAB Function5/1(t), MATLAB Function4/2(t)
  Subsystem3/1(Threshold) -> Subtract2/2, Scope9/2, Subtract3/2, threshold_view/1
  neuron_num/1 -> Subsystem3/3(neuron_num)
  From Workspace4/1 -> Subsystem3/2(initial_threshold)
  MATLAB Function5/1(membrane_potential) -> Scope4/4, Switch1/1
  MATLAB Function4/1(membrane_potential) -> Switch1/3, Scope4/5
  Subsystem2/1(membrane_state) -> MATLAB Function4/1(membrane_state), Subtract3/1, Scope4/2, MATLAB Function5/2(membrane_state)
  spike_generator1/1(spike) -> "Spike "/1, Scope9/6, Subsystem3/1(spike)
  Input_potential/1 -> Subsystem2/1(Input potential), Subsystem2/Trigger, Scope4/1, Clock4/2("Reset ")
  Subtract3/1 -> Switch1/2
  Memory2/1 -> Scope9/5, spike_generator1/1(1)
  Delay/1 -> Subsystem2/2(before_Potential)
  clock/1 -> Subsystem3/4(clock), Clock4/1(clock)

== system pattern3x3_training_2023clock/Neuron8 ==
  note: Membrane potential part
  note: Input potential이 추가로 들어오기 전에는 이전
      | membrane state를 유지해야 하기 때문에 Trigger 사용
  note: Output 스파이크 빈도에 따라 Threshold 조절
  note: membrane potential>=threshold
  note: membrane potential
      | - threshold
  note: 뉴런 번호
  note: membrane potential<threshold
  note: membrane potential - threshold >= 0 일때 spike=1
  note: Threshold part
  note: Spike part
  note: membrane state
      | - threshold
  clock : Inport
  Input_potential : Inport  Port=2  OutDataTypeStr=double
  neuron_num : Inport  Port=3  OutDataTypeStr=double
  Clock4 : Subsystem
  Delay : Delay  DelayLength=1  InitialCondition=0
  From Workspace4 : FromWorkspace  VariableName=threshold_pre
  MATLAB Function3 : MATLAB Function  TreatAsAtomicUnit=on
  MATLAB Function4 : MATLAB Function  TreatAsAtomicUnit=on
  MATLAB Function5 : MATLAB Function  TreatAsAtomicUnit=on
  Memory2 : Memory
  Scope4 : Scope  NumInputPorts=5
  Scope9 : Scope  NumInputPorts=6
  Subsystem2 : Subsystem
  Subsystem3 : Subsystem
  Subtract2 : Sum  Inputs=+-
  Subtract3 : Sum  Inputs=+-
  Switch1 : Switch  SaturateOnIntegerOverflow=off  InputSameDT=off
  spike_generator1 : Subsystem
  "Spike " : Outport  VectorParamsAs1DForOutWhenUnconnected=off
  threshold_view : Outport  Port=2
  wires:
  Switch1/1 -> Delay/1, Subtract2/1, Scope9/1
  Subtract2/1 -> Scope9/3, MATLAB Function3/1(u)
  MATLAB Function3/1(y) -> Memory2/1, Scope9/4
  Clock4/1(T) -> Scope4/3, MATLAB Function5/1(t), MATLAB Function4/2(t)
  Subsystem3/1(Threshold) -> Subtract2/2, Scope9/2, Subtract3/2, threshold_view/1
  neuron_num/1 -> Subsystem3/3(neuron_num)
  From Workspace4/1 -> Subsystem3/2(initial_threshold)
  MATLAB Function5/1(membrane_potential) -> Scope4/4, Switch1/1
  MATLAB Function4/1(membrane_potential) -> Switch1/3, Scope4/5
  Subsystem2/1(membrane_state) -> MATLAB Function4/1(membrane_state), Subtract3/1, Scope4/2, MATLAB Function5/2(membrane_state)
  spike_generator1/1(spike) -> "Spike "/1, Scope9/6, Subsystem3/1(spike)
  Input_potential/1 -> Subsystem2/1(Input potential), Subsystem2/Trigger, Scope4/1, Clock4/2("Reset ")
  Subtract3/1 -> Switch1/2
  Memory2/1 -> Scope9/5, spike_generator1/1(1)
  Delay/1 -> Subsystem2/2(before_Potential)
  clock/1 -> Subsystem3/4(clock), Clock4/1(clock)

== system pattern3x3_training_2023clock/Neuron9 ==
  note: Membrane potential part
  note: Input potential이 추가로 들어오기 전에는 이전
      | membrane state를 유지해야 하기 때문에 Trigger 사용
  note: Output 스파이크 빈도에 따라 Threshold 조절
  note: membrane potential>=threshold
  note: membrane potential
      | - threshold
  note: 뉴런 번호
  note: membrane potential<threshold
  note: membrane potential - threshold >= 0 일때 spike=1
  note: Threshold part
  note: Spike part
  note: membrane state
      | - threshold
  clock : Inport
  Input_potential : Inport  Port=2  OutDataTypeStr=double
  neuron_num : Inport  Port=3  OutDataTypeStr=double
  Clock4 : Subsystem
  Delay : Delay  DelayLength=1  InitialCondition=0
  From Workspace4 : FromWorkspace  VariableName=threshold_pre
  MATLAB Function3 : MATLAB Function  TreatAsAtomicUnit=on
  MATLAB Function4 : MATLAB Function  TreatAsAtomicUnit=on
  MATLAB Function5 : MATLAB Function  TreatAsAtomicUnit=on
  Memory2 : Memory
  Scope4 : Scope  NumInputPorts=5
  Scope9 : Scope  NumInputPorts=6
  Subsystem2 : Subsystem
  Subsystem3 : Subsystem
  Subtract2 : Sum  Inputs=+-
  Subtract3 : Sum  Inputs=+-
  Switch1 : Switch  SaturateOnIntegerOverflow=off  InputSameDT=off
  spike_generator1 : Subsystem
  "Spike " : Outport  VectorParamsAs1DForOutWhenUnconnected=off
  threshold_view : Outport  Port=2
  wires:
  Switch1/1 -> Delay/1, Subtract2/1, Scope9/1
  Subtract2/1 -> Scope9/3, MATLAB Function3/1(u)
  MATLAB Function3/1(y) -> Memory2/1, Scope9/4
  Clock4/1(T) -> Scope4/3, MATLAB Function5/1(t), MATLAB Function4/2(t)
  Subsystem3/1(Threshold) -> Subtract2/2, Scope9/2, Subtract3/2, threshold_view/1
  neuron_num/1 -> Subsystem3/3(neuron_num)
  From Workspace4/1 -> Subsystem3/2(initial_threshold)
  MATLAB Function5/1(membrane_potential) -> Scope4/4, Switch1/1
  MATLAB Function4/1(membrane_potential) -> Switch1/3, Scope4/5
  Subsystem2/1(membrane_state) -> MATLAB Function4/1(membrane_state), Subtract3/1, Scope4/2, MATLAB Function5/2(membrane_state)
  spike_generator1/1(spike) -> "Spike "/1, Scope9/6, Subsystem3/1(spike)
  Input_potential/1 -> Subsystem2/1(Input potential), Subsystem2/Trigger, Scope4/1, Clock4/2("Reset ")
  Subtract3/1 -> Switch1/2
  Memory2/1 -> Scope9/5, spike_generator1/1(1)
  Delay/1 -> Subsystem2/2(before_Potential)
  clock/1 -> Subsystem3/4(clock), Clock4/1(clock)

== system pattern3x3_training_2023clock/Post_Neuron1 ==
  note: 측면 억제로 다른 post 뉴런이 발화하면 membrane potential을 낮춘다
  clock : Inport
  Input_potential : Inport  Port=2  OutDataTypeStr=double
  neuron_num : Inport  Port=3  OutDataTypeStr=double
  wta : Inport  Port=4
  Clock1 : Subsystem
  Clock2 : Subsystem
  Delay : Delay  DelayLength=1  InitialCondition=0
  From Workspace4 : FromWorkspace  VariableName=threshold_post
  From Workspace6 : FromWorkspace  VariableName=later_table
  From Workspace7 : FromWorkspace  VariableName=inhibition_rc
  MATLAB Function1 : MATLAB Function  TreatAsAtomicUnit=on
  MATLAB Function2 : MATLAB Function  TreatAsAtomicUnit=on
  MATLAB Function3 : MATLAB Function  TreatAsAtomicUnit=on
  MATLAB Function4 : MATLAB Function  TreatAsAtomicUnit=on
  MATLAB Function7 : MATLAB Function  TreatAsAtomicUnit=on
  Product : Product
  Scope{1,3..4,9} (4 alike) : Scope  NumInputPorts=4
  Subsystem1 : Subsystem
  Subsystem3 : Subsystem
  Subtract2 : Sum  Inputs=++-
  Subtract3 : Sum  Inputs=++-
  Switch1 : Switch  SaturateOnIntegerOverflow=off  InputSameDT=off
  memory : Subsystem
  spike_generator1 : Subsystem
  Spike : Outport  VectorParamsAs1DForOutWhenUnconnected=off
  threshold_view : Outport  Port=2
  wires:
  MATLAB Function4/1(membrane_potential) -> Scope3/3, Switch1/1
  Clock1/1(T) -> MATLAB Function4/1(t), MATLAB Function3/2(t)
  From Workspace4/1 -> Subsystem3/2(initial_threshold)
  neuron_num/1 -> Subsystem3/3(neuron_num)
  Input_potential/1 -> Subsystem1/1(In1), Subsystem1/Trigger, Clock1/2("Reset "), Scope3/1
  Subsystem1/1(membrane_state) -> MATLAB Function3/1(membrane_state), Subtract2/1, MATLAB Function4/2(membrane_state), Scope3/2
  Subtract2/1 -> Switch1/2
  Subsystem3/1(Threshold) -> Subtract3/3, Subtract2/3, threshold_view/1
  wta/1 -> Clock2/2("Reset "), Scope4/1, MATLAB Function2/1(u), Scope1/2
  MATLAB Function3/1(membrane_potential) -> Switch1/3, Scope3/4
  Clock2/1(T) -> MATLAB Function7/3(t)
  From Workspace6/1 -> MATLAB Function7/2(lateral_inhibition)
  Product/1 -> Subtract2/2, Scope1/3, Subtract3/2, Scope4/2
  From Workspace7/1 -> MATLAB Function7/1(rc)
  memory/1(Out1) -> Scope9/3, spike_generator1/1(1)
  MATLAB Function1/1(y) -> memory/1(In1), Scope9/2
  spike_generator1/1(spike) -> Scope9/4, Spike/1, Scope1/1, Subsystem3/1(spike)
  Subtract3/1 -> Scope1/4, Scope4/4, MATLAB Function1/1(u), Scope9/1
  Switch1/1 -> Subtract3/1, Delay/1, Scope4/3
  MATLAB Function2/1(y) -> Product/2
  MATLAB Function7/1(inhibition_potential) -> Product/1
  Delay/1 -> Subsystem1/2(In2)
  clock/1 -> Clock2/1(clock), Subsystem3/4(clock), Clock1/1(clock)

== system pattern3x3_training_2023clock/Post_Neuron2 ==
  note: 측면 억제로 다른 post 뉴런이 발화하면 membrane potential을 낮춘다
  clock : Inport
  Input_potential : Inport  Port=2  OutDataTypeStr=double
  neuron_num : Inport  Port=3  OutDataTypeStr=double
  wta : Inport  Port=4
  Clock1 : Subsystem
  Clock2 : Subsystem
  Delay : Delay  DelayLength=1  InitialCondition=0
  From Workspace4 : FromWorkspace  VariableName=threshold_post
  From Workspace6 : FromWorkspace  VariableName=later_table
  From Workspace7 : FromWorkspace  VariableName=inhibition_rc
  MATLAB Function1 : MATLAB Function  TreatAsAtomicUnit=on
  MATLAB Function2 : MATLAB Function  TreatAsAtomicUnit=on
  MATLAB Function3 : MATLAB Function  TreatAsAtomicUnit=on
  MATLAB Function4 : MATLAB Function  TreatAsAtomicUnit=on
  MATLAB Function7 : MATLAB Function  TreatAsAtomicUnit=on
  Product : Product
  Scope{1,3..4,9} (4 alike) : Scope  NumInputPorts=4
  Subsystem1 : Subsystem
  Subsystem3 : Subsystem
  Subtract2 : Sum  Inputs=++-
  Subtract3 : Sum  Inputs=++-
  Switch1 : Switch  SaturateOnIntegerOverflow=off  InputSameDT=off
  memory : Subsystem
  spike_generator1 : Subsystem
  Spike : Outport  VectorParamsAs1DForOutWhenUnconnected=off
  threshold_view : Outport  Port=2
  wires:
  MATLAB Function4/1(membrane_potential) -> Scope3/3, Switch1/1
  Clock1/1(T) -> MATLAB Function4/1(t), MATLAB Function3/2(t)
  From Workspace4/1 -> Subsystem3/2(initial_threshold)
  neuron_num/1 -> Subsystem3/3(neuron_num)
  Input_potential/1 -> Subsystem1/1(In1), Subsystem1/Trigger, Clock1/2("Reset "), Scope3/1
  Subsystem1/1(membrane_state) -> MATLAB Function3/1(membrane_state), Subtract2/1, MATLAB Function4/2(membrane_state), Scope3/2
  Subtract2/1 -> Switch1/2
  Subsystem3/1(Threshold) -> Subtract3/3, Subtract2/3, threshold_view/1
  wta/1 -> Clock2/2("Reset "), Scope4/1, MATLAB Function2/1(u), Scope1/2
  MATLAB Function3/1(membrane_potential) -> Switch1/3, Scope3/4
  Clock2/1(T) -> MATLAB Function7/3(t)
  From Workspace6/1 -> MATLAB Function7/2(lateral_inhibition)
  Product/1 -> Subtract2/2, Scope1/3, Subtract3/2, Scope4/2
  From Workspace7/1 -> MATLAB Function7/1(rc)
  memory/1(Out1) -> Scope9/3, spike_generator1/1(1)
  MATLAB Function1/1(y) -> memory/1(In1), Scope9/2
  spike_generator1/1(spike) -> Scope9/4, Spike/1, Scope1/1, Subsystem3/1(spike)
  Subtract3/1 -> Scope1/4, Scope4/4, MATLAB Function1/1(u), Scope9/1
  Switch1/1 -> Subtract3/1, Delay/1, Scope4/3
  MATLAB Function2/1(y) -> Product/2
  MATLAB Function7/1(inhibition_potential) -> Product/1
  Delay/1 -> Subsystem1/2(In2)
  clock/1 -> Clock2/1(clock), Subsystem3/4(clock), Clock1/1(clock)

== system pattern3x3_training_2023clock/Post_Neuron3 ==
  note: 측면 억제로 다른 post 뉴런이 발화하면 membrane potential을 낮춘다
  clock : Inport
  Input_potential : Inport  Port=2  OutDataTypeStr=double
  neuron_num : Inport  Port=3  OutDataTypeStr=double
  wta : Inport  Port=4
  Clock1 : Subsystem
  Clock2 : Subsystem
  Delay : Delay  DelayLength=1  InitialCondition=0
  From Workspace4 : FromWorkspace  VariableName=threshold_post
  From Workspace6 : FromWorkspace  VariableName=later_table
  From Workspace7 : FromWorkspace  VariableName=inhibition_rc
  MATLAB Function1 : MATLAB Function  TreatAsAtomicUnit=on
  MATLAB Function2 : MATLAB Function  TreatAsAtomicUnit=on
  MATLAB Function3 : MATLAB Function  TreatAsAtomicUnit=on
  MATLAB Function4 : MATLAB Function  TreatAsAtomicUnit=on
  MATLAB Function7 : MATLAB Function  TreatAsAtomicUnit=on
  Product : Product
  Scope{1,3..4,9} (4 alike) : Scope  NumInputPorts=4
  Subsystem1 : Subsystem
  Subsystem3 : Subsystem
  Subtract2 : Sum  Inputs=++-
  Subtract3 : Sum  Inputs=++-
  Switch1 : Switch  SaturateOnIntegerOverflow=off  InputSameDT=off
  memory : Subsystem
  spike_generator1 : Subsystem
  Spike : Outport  VectorParamsAs1DForOutWhenUnconnected=off
  threshold_view : Outport  Port=2
  wires:
  MATLAB Function4/1(membrane_potential) -> Scope3/3, Switch1/1
  Clock1/1(T) -> MATLAB Function4/1(t), MATLAB Function3/2(t)
  From Workspace4/1 -> Subsystem3/2(initial_threshold)
  neuron_num/1 -> Subsystem3/3(neuron_num)
  Input_potential/1 -> Subsystem1/1(In1), Subsystem1/Trigger, Clock1/2("Reset "), Scope3/1
  Subsystem1/1(membrane_state) -> MATLAB Function3/1(membrane_state), Subtract2/1, MATLAB Function4/2(membrane_state), Scope3/2
  Subtract2/1 -> Switch1/2
  Subsystem3/1(Threshold) -> Subtract3/3, Subtract2/3, threshold_view/1
  wta/1 -> Clock2/2("Reset "), Scope4/1, MATLAB Function2/1(u), Scope1/2
  MATLAB Function3/1(membrane_potential) -> Switch1/3, Scope3/4
  Clock2/1(T) -> MATLAB Function7/3(t)
  From Workspace6/1 -> MATLAB Function7/2(lateral_inhibition)
  Product/1 -> Subtract2/2, Scope1/3, Subtract3/2, Scope4/2
  From Workspace7/1 -> MATLAB Function7/1(rc)
  memory/1(Out1) -> Scope9/3, spike_generator1/1(1)
  MATLAB Function1/1(y) -> memory/1(In1), Scope9/2
  spike_generator1/1(spike) -> Scope9/4, Spike/1, Scope1/1, Subsystem3/1(spike)
  Subtract3/1 -> Scope1/4, Scope4/4, MATLAB Function1/1(u), Scope9/1
  Switch1/1 -> Subtract3/1, Delay/1, Scope4/3
  MATLAB Function2/1(y) -> Product/2
  MATLAB Function7/1(inhibition_potential) -> Product/1
  Delay/1 -> Subsystem1/2(In2)
  clock/1 -> Clock2/1(clock), Subsystem3/4(clock), Clock1/1(clock)
